simulink model "OPENXWD"  (R2022b)
settings: Solver=ode45  StartTime=0.0  StopTime=inf  RelTol=1e-3  EnableMultiTasking=on
PreLoadFcn:
  | run('Parameters\FSE_Parameters.m')
values from neighbouring files (symbols this model uses):
  g = 9.81    [script.m]    (also in srcipt.m)
  h = 0.25    [script.m]    (also in srcipt.m)
  Ki_pl = 0.01    [srcipt.m]
  Kp_pl = 0.1    [srcipt.m]
  L = 2.6    [script.m]    (also in srcipt.m)
  lf = 2.1    [script.m]    (also in srcipt.m)
  lr = 0.5    [script.m]    (also in srcipt.m)
  ls = 1.242    [script.m]    (also in srcipt.m)
  m = 180    [script.m]    (also in srcipt.m)
  rw = 0.217    [script.m]    (also in srcipt.m)
  Ts = 0.01    [srcipt.m]
undefined symbols (not defined in the file or in its folder): c, gain, Ku, l_ESO, min_yaw_rate
libraries: CarMaker4SL x45, simulink x9
(part 3 of 3)

== system OPENXWD/CarMaker/IPG Vehicle/PowerTrain/TorqueVectoring/Torque distribution/T_FR1 ==
  FzRR : Inport
  Tt : Inport  Port=2
  ^Mz : Inport  Port=3
  Gain : Gain  Gain=rw/ls
  Gain1 : Gain  Gain=1/(m*g)
  Product : Product
  Sum : Sum
  T_RR : Outport
  wires:
  Gain/1 -> Sum/2
  Tt/1 -> Sum/1
  ^Mz/1 -> Gain/1
  FzRR/1 -> Gain1/1
  Gain1/1 -> Product/1
  Product/1 -> T_RR/1
  Sum/1 -> Product/2

== system OPENXWD/CarMaker/IPG Vehicle/PowerTrain/TorqueVectoring/Torque distribution/T_RL ==
  FzRL : Inport
  Tt : Inport  Port=2
  ^Mz : Inport  Port=3
  Gain : Gain  Gain=rw/ls
  Gain1 : Gain  Gain=1/(m*g)
  Product : Product
  Sum : Sum  Inputs=+-
  T_RL : Outport
  wires:
  Gain/1 -> Sum/2
  Tt/1 -> Sum/1
  ^Mz/1 -> Gain/1
  FzRL/1 -> Gain1/1
  Gain1/1 -> Product/1
  Product/1 -> T_RL/1
  Sum/1 -> Product/2

== system OPENXWD/CarMaker/IPG Vehicle/TV/TorqueVectoring/Torque distribution/Fzfl ==
  ax : Inport
  ay : Inport  Port=2
  Constant : Constant  Value=g*lr
  Gain : Gain  Gain=m/(2*L)
  Gain1 : Gain  Gain=h
  Gain2 : Gain  Gain=(h*lr)/(ls)
  Sum : Sum  Inputs=+--
  Fzfl : Outport
  wires:
  Sum/1 -> Gain/1
  Constant/1 -> Sum/1
  Gain1/1 -> Sum/2
  ax/1 -> Gain1/1
  ay/1 -> Gain2/1
  Gain2/1 -> Sum/3
  Gain/1 -> Fzfl/1

== system OPENXWD/CarMaker/IPG Vehicle/TV/TorqueVectoring/Torque distribution/Fzfr ==
  ay : Inport
  ax : Inport  Port=2
  Constant : Constant  Value=g*lr
  Gain : Gain  Gain=m/(2*L)
  Gain1 : Gain  Gain=h
  Gain2 : Gain  Gain=(h*lr)/(ls)
  Sum : Sum  Inputs=+-+
  Fzfr : Outport
  wires:
  Sum/1 -> Gain/1
  Constant/1 -> Sum/1
  Gain1/1 -> Sum/2
  ax/1 -> Gain1/1
  ay/1 -> Gain2/1
  Gain2/1 -> Sum/3
  Gain/1 -> Fzfr/1

== system OPENXWD/CarMaker/IPG Vehicle/TV/TorqueVectoring/Torque distribution/Fzrl ==
  ax : Inport
  ay : Inport  Port=2
  Constant : Constant  Value=g*lf
  Gain : Gain  Gain=m/(2*L)
  Gain1 : Gain  Gain=h
  Gain2 : Gain  Gain=(h*lf)/(ls)
  Sum : Sum  Inputs=++-
  Fzrl : Outport
  wires:
  Gain/1 -> Fzrl/1
  Gain2/1 -> Sum/3
  ay/1 -> Gain2/1
  Sum/1 -> Gain/1
  Constant/1 -> Sum/1
  ax/1 -> Gain1/1
  Gain1/1 -> Sum/2

== system OPENXWD/CarMaker/IPG Vehicle/TV/TorqueVectoring/Torque distribution/Fzrr ==
  ay : Inport
  ax : Inport  Port=2
  Constant : Constant  Value=g*lf
  Gain : Gain  Gain=m/(2*L)
  Gain1 : Gain  Gain=h
  Gain2 : Gain  Gain=(h*lf)/(ls)
  Sum : Sum  Inputs=+++
  Fzrr : Outport
  wires:
  Gain/1 -> Fzrr/1
  Gain2/1 -> Sum/3
  ay/1 -> Gain2/1
  Sum/1 -> Gain/1
  Constant/1 -> Sum/1
  ax/1 -> Gain1/1
  Gain1/1 -> Sum/2

== system OPENXWD/CarMaker/IPG Vehicle/TV/TorqueVectoring/Torque distribution/Regulator ==
  User input : Inport
  Rear wheels speed : Inport  Port=2
  Vehicle speed : Inport  Port=3
  Constant : Constant  Value=0.1175
  Constant1 : Constant  Value=0
  Feedback controler : Subsystem
  Govenor : Subsystem
  Power Limiting : Subsystem
  Saturation Dynamic : simulink/Discontinuities/Saturation Dynamic  OutMin=[]  OutMax=[]  OutDataTypeStr=Inherit: Same as second input  OutDataType=fixdt(1, 16)  OutScaling=2^-10  DoSatur=off
  Sum : Sum  Inputs=|+-
  Zero-Order Hold : ZeroOrderHold  SampleTime=c.Ts
  demanded torque : Outport
  wires:
  Zero-Order Hold/1 -> Feedback controler/1(e)
  Rear wheels speed/1 -> Power Limiting/1(rear wheel speed), Sum/2  "rear_wheel_speed[m/s]"
  Sum/1 -> Zero-Order Hold/1  "e_wheels_speed[m/s]"
  Constant/1 -> Govenor/1(Ref slip ratio)
  Govenor/1(velocity) -> Sum/1  "ref_v_R [m/s]"
  User input/1 -> Feedback controler/2(User input)
  Vehicle speed/1 -> Govenor/2(vehicle speed)
  Saturation Dynamic/1 -> demanded torque/1, Feedback controler/3(u_now)
  Feedback controler/1(demanded torque) -> Saturation Dynamic/2
  Constant1/1 -> Saturation Dynamic/3
  Power Limiting/1(Out1) -> Saturation Dynamic/1  "torque_power_limiting[Nm]"

== system OPENXWD/CarMaker/IPG Vehicle/TV/TorqueVectoring/Torque distribution/Regulator1 ==
  User input : Inport
  Rear wheels speed : Inport  Port=2
  Vehicle speed : Inport  Port=3
  Constant : Constant  Value=0.1175
  Constant1 : Constant  Value=0
  Feedback controler : Subsystem
  Govenor : Subsystem
  Power Limiting : Subsystem
  Saturation Dynamic : simulink/Discontinuities/Saturation Dynamic  OutMin=[]  OutMax=[]  OutDataTypeStr=Inherit: Same as second input  OutDataType=fixdt(1, 16)  OutScaling=2^-10  DoSatur=off
  Sum : Sum  Inputs=|+-
  Zero-Order Hold : ZeroOrderHold  SampleTime=c.Ts
  demanded torque : Outport
  wires:
  Zero-Order Hold/1 -> Feedback controler/1(e)
  Rear wheels speed/1 -> Power Limiting/1(rear wheel speed), Sum/2  "rear_wheel_speed[m/s]"
  Sum/1 -> Zero-Order Hold/1  "e_wheels_speed[m/s]"
  Constant/1 -> Govenor/1(Ref slip ratio)
  Govenor/1(velocity) -> Sum/1  "ref_v_R [m/s]"
  User input/1 -> Feedback controler/2(User input)
  Vehicle speed/1 -> Govenor/2(vehicle speed)
  Saturation Dynamic/1 -> demanded torque/1, Feedback controler/3(u_now)
  Feedback controler/1(demanded torque) -> Saturation Dynamic/2
  Constant1/1 -> Saturation Dynamic/3
  Power Limiting/1(Out1) -> Saturation Dynamic/1  "torque_power_limiting[Nm]"

== system OPENXWD/CarMaker/IPG Vehicle/TV/TorqueVectoring/Torque distribution/Regulator2 ==
  User input : Inport
  Rear wheels speed : Inport  Port=2
  Vehicle speed : Inport  Port=3
  Constant : Constant  Value=0.1175
  Constant1 : Constant  Value=0
  Feedback controler : Subsystem
  Govenor : Subsystem
  Power Limiting : Subsystem
  Saturation Dynamic : simulink/Discontinuities/Saturation Dynamic  OutMin=[]  OutMax=[]  OutDataTypeStr=Inherit: Same as second input  OutDataType=fixdt(1, 16)  OutScaling=2^-10  DoSatur=off
  Sum : Sum  Inputs=|+-
  Zero-Order Hold : ZeroOrderHold  SampleTime=c.Ts
  demanded torque : Outport
  wires:
  Zero-Order Hold/1 -> Feedback controler/1(e)
  Rear wheels speed/1 -> Power Limiting/1(rear wheel speed), Sum/2  "rear_wheel_speed[m/s]"
  Sum/1 -> Zero-Order Hold/1  "e_wheels_speed[m/s]"
  Constant/1 -> Govenor/1(Ref slip ratio)
  Govenor/1(velocity) -> Sum/1  "ref_v_R [m/s]"
  User input/1 -> Feedback controler/2(User input)
  Vehicle speed/1 -> Govenor/2(vehicle speed)
  Saturation Dynamic/1 -> demanded torque/1, Feedback controler/3(u_now)
  Feedback controler/1(demanded torque) -> Saturation Dynamic/2
  Constant1/1 -> Saturation Dynamic/3
  Power Limiting/1(Out1) -> Saturation Dynamic/1  "torque_power_limiting[Nm]"

== system OPENXWD/CarMaker/IPG Vehicle/TV/TorqueVectoring/Torque distribution/Regulator3 ==
  User input : Inport
  Rear wheels speed : Inport  Port=2
  Vehicle speed : Inport  Port=3
  Constant : Constant  Value=0.1175
  Constant1 : Constant  Value=0
  Feedback controler : Subsystem
  Govenor : Subsystem
  Power Limiting : Subsystem
  Saturation Dynamic : simulink/Discontinuities/Saturation Dynamic  OutMin=[]  OutMax=[]  OutDataTypeStr=Inherit: Same as second input  OutDataType=fixdt(1, 16)  OutScaling=2^-10  DoSatur=off
  Sum : Sum  Inputs=|+-
  Zero-Order Hold : ZeroOrderHold  SampleTime=c.Ts
  demanded torque : Outport
  wires:
  Zero-Order Hold/1 -> Feedback controler/1(e)
  Rear wheels speed/1 -> Power Limiting/1(rear wheel speed), Sum/2  "rear_wheel_speed[m/s]"
  Sum/1 -> Zero-Order Hold/1  "e_wheels_speed[m/s]"
  Constant/1 -> Govenor/1(Ref slip ratio)
  Govenor/1(velocity) -> Sum/1  "ref_v_R [m/s]"
  User input/1 -> Feedback controler/2(User input)
  Vehicle speed/1 -> Govenor/2(vehicle speed)
  Saturation Dynamic/1 -> demanded torque/1, Feedback controler/3(u_now)
  Feedback controler/1(demanded torque) -> Saturation Dynamic/2
  Constant1/1 -> Saturation Dynamic/3
  Power Limiting/1(Out1) -> Saturation Dynamic/1  "torque_power_limiting[Nm]"

== system OPENXWD/CarMaker/IPG Vehicle/TV/TorqueVectoring/Torque distribution/T_FL ==
  Fzfl : Inport
  Tt : Inport  Port=2
  ^Mz : Inport  Port=3
  Gain : Gain  Gain=rw/ls
  Gain1 : Gain  Gain=1/(m*g)
  Product : Product
  Sum : Sum  Inputs=+-
  T_FL : Outport
  wires:
  Gain/1 -> Sum/2
  Tt/1 -> Sum/1
  ^Mz/1 -> Gain/1
  Fzfl/1 -> Gain1/1
  Gain1/1 -> Product/1
  Product/1 -> T_FL/1
  Sum/1 -> Product/2

== system OPENXWD/CarMaker/IPG Vehicle/TV/TorqueVectoring/Torque distribution/T_FR ==
  Fzfr : Inport
  Tt : Inport  Port=2
  ^Mz : Inport  Port=3
  Gain : Gain  Gain=rw/ls
  Gain1 : Gain  Gain=1/(m*g)
  Product : Product
  Sum : Sum
  T_FR : Outport
  wires:
  Gain/1 -> Sum/2
  Tt/1 -> Sum/1
  ^Mz/1 -> Gain/1
  Fzfr/1 -> Gain1/1
  Gain1/1 -> Product/1
  Product/1 -> T_FR/1
  Sum/1 -> Product/2

== system OPENXWD/CarMaker/IPG Vehicle/TV/TorqueVectoring/Torque distribution/T_RL ==
  FzRL : Inport
  Tt : Inport  Port=2
  ^Mz : Inport  Port=3
  Gain : Gain  Gain=rw/ls
  Gain1 : Gain  Gain=1/(m*g)
  Product : Product
  Sum : Sum  Inputs=+-
  T_RL : Outport
  wires:
  Gain/1 -> Sum/2
  Tt/1 -> Sum/1
  ^Mz/1 -> Gain/1
  FzRL/1 -> Gain1/1
  Gain1/1 -> Product/1
  Product/1 -> T_RL/1
  Sum/1 -> Product/2

== system OPENXWD/CarMaker/IPG Vehicle/TV/TorqueVectoring/Torque distribution/T_RR ==
  FzRR : Inport
  Tt : Inport  Port=2
  ^Mz : Inport  Port=3
  Gain : Gain  Gain=rw/ls
  Gain1 : Gain  Gain=1/(m*g)
  Product : Product
  Sum : Sum
  T_RR : Outport
  wires:
  Gain/1 -> Sum/2
  Tt/1 -> Sum/1
  ^Mz/1 -> Gain/1
  FzRR/1 -> Gain1/1
  Gain1/1 -> Product/1
  Product/1 -> T_RR/1
  Sum/1 -> Product/2

== system OPENXWD/CarMaker/IPG Vehicle/The Best TorqueVectoring/TorqueVectoring/Torque distribution Tv/Fzfl ==
  ax : Inport
  ay : Inport  Port=2
  Constant : Constant  Value=g*lr
  Gain : Gain  Gain=m/(2*L)
  Gain1 : Gain  Gain=h
  Gain2 : Gain  Gain=(h*lr)/(ls)
  Sum : Sum  Inputs=+--
  Fzfl : Outport
  wires:
  Sum/1 -> Gain/1
  Constant/1 -> Sum/1
  Gain1/1 -> Sum/2
  ax/1 -> Gain1/1
  ay/1 -> Gain2/1
  Gain2/1 -> Sum/3
  Gain/1 -> Fzfl/1

== system OPENXWD/CarMaker/IPG Vehicle/The Best TorqueVectoring/TorqueVectoring/Torque distribution Tv/Fzfr ==
  ay : Inport
  ax : Inport  Port=2
  Constant : Constant  Value=g*lr
  Gain : Gain  Gain=m/(2*L)
  Gain1 : Gain  Gain=h
  Gain2 : Gain  Gain=(h*lr)/(ls)
  Sum : Sum  Inputs=+-+
  Fzfr : Outport
  wires:
  Sum/1 -> Gain/1
  Constant/1 -> Sum/1
  Gain1/1 -> Sum/2
  ax/1 -> Gain1/1
  ay/1 -> Gain2/1
  Gain2/1 -> Sum/3
  Gain/1 -> Fzfr/1

== system OPENXWD/CarMaker/IPG Vehicle/The Best TorqueVectoring/TorqueVectoring/Torque distribution Tv/Fzrl ==
  ax : Inport
  ay : Inport  Port=2
  Constant : Constant  Value=g*lf
  Gain : Gain  Gain=m/(2*L)
  Gain1 : Gain  Gain=h
  Gain2 : Gain  Gain=(h*lf)/(ls)
  Sum : Sum  Inputs=++-
  Fzrl : Outport
  wires:
  Gain/1 -> Fzrl/1
  Gain2/1 -> Sum/3
  ay/1 -> Gain2/1
  Sum/1 -> Gain/1
  Constant/1 -> Sum/1
  ax/1 -> Gain1/1
  Gain1/1 -> Sum/2

== system OPENXWD/CarMaker/IPG Vehicle/The Best TorqueVectoring/TorqueVectoring/Torque distribution Tv/Fzrr ==
  ay : Inport
  ax : Inport  Port=2
  Constant : Constant  Value=g*lf
  Gain : Gain  Gain=m/(2*L)
  Gain1 : Gain  Gain=h
  Gain2 : Gain  Gain=(h*lf)/(ls)
  Sum : Sum  Inputs=+++
  Fzrr : Outport
  wires:
  Gain/1 -> Fzrr/1
  Gain2/1 -> Sum/3
  ay/1 -> Gain2/1
  Sum/1 -> Gain/1
  Constant/1 -> Sum/1
  ax/1 -> Gain1/1
  Gain1/1 -> Sum/2

== system OPENXWD/CarMaker/IPG Vehicle/The Best TorqueVectoring/TorqueVectoring/Torque distribution Tv/T_FL ==
  Fzfl : Inport
  Tt : Inport  Port=2
  ^Mz : Inport  Port=3
  Gain : Gain  Gain=rw/ls
  Gain1 : Gain  Gain=1/(m*g)
  Product : Product
  Sum : Sum  Inputs=+-
  T_FL : Outport
  wires:
  Gain/1 -> Sum/2
  Tt/1 -> Sum/1
  ^Mz/1 -> Gain/1
  Fzfl/1 -> Gain1/1
  Gain1/1 -> Product/1
  Product/1 -> T_FL/1
  Sum/1 -> Product/2

== system OPENXWD/CarMaker/IPG Vehicle/The Best TorqueVectoring/TorqueVectoring/Torque distribution Tv/T_FR ==
  Fzfr : Inport
  Tt : Inport  Port=2
  ^Mz : Inport  Port=3
  Gain : Gain  Gain=rw/ls
  Gain1 : Gain  Gain=1/(m*g)
  Product : Product
  Sum : Sum
  T_FR : Outport
  wires:
  Gain/1 -> Sum/2
  Tt/1 -> Sum/1
  ^Mz/1 -> Gain/1
  Fzfr/1 -> Gain1/1
  Gain1/1 -> Product/1
  Product/1 -> T_FR/1
  Sum/1 -> Product/2

== system OPENXWD/CarMaker/IPG Vehicle/The Best TorqueVectoring/TorqueVectoring/Torque distribution Tv/T_FR1 ==
  FzRR : Inport
  Tt : Inport  Port=2
  ^Mz : Inport  Port=3
  Gain : Gain  Gain=rw/ls
  Gain1 : Gain  Gain=1/(m*g)
  Product : Product
  Sum : Sum
  T_RR : Outport
  wires:
  Gain/1 -> Sum/2
  Tt/1 -> Sum/1
  ^Mz/1 -> Gain/1
  FzRR/1 -> Gain1/1
  Gain1/1 -> Product/1
  Product/1 -> T_RR/1
  Sum/1 -> Product/2

== system OPENXWD/CarMaker/IPG Vehicle/The Best TorqueVectoring/TorqueVectoring/Torque distribution Tv/T_RL ==
  FzRL : Inport
  Tt : Inport  Port=2
  ^Mz : Inport  Port=3
  Gain : Gain  Gain=rw/ls
  Gain1 : Gain  Gain=1/(m*g)
  Product : Product
  Sum : Sum  Inputs=+-
  T_RL : Outport
  wires:
  Gain/1 -> Sum/2
  Tt/1 -> Sum/1
  ^Mz/1 -> Gain/1
  FzRL/1 -> Gain1/1
  Gain1/1 -> Product/1
  Product/1 -> T_RL/1
  Sum/1 -> Product/2

== system OPENXWD/CarMaker/IPG Vehicle/TorqueVectoring/TorqueVectoring/Torque distribution/Fzfl ==
  ax : Inport
  ay : Inport  Port=2
  Constant : Constant  Value=g*lr
  Gain : Gain  Gain=m/(2*L)
  Gain1 : Gain  Gain=h
  Gain2 : Gain  Gain=(h*lr)/(ls)
  Sum : Sum  Inputs=+--
  Fzfl : Outport
  wires:
  Sum/1 -> Gain/1
  Constant/1 -> Sum/1
  Gain1/1 -> Sum/2
  ax/1 -> Gain1/1
  ay/1 -> Gain2/1
  Gain2/1 -> Sum/3
  Gain/1 -> Fzfl/1

== system OPENXWD/CarMaker/IPG Vehicle/TorqueVectoring/TorqueVectoring/Torque distribution/Fzfr ==
  ay : Inport
  ax : Inport  Port=2
  Constant : Constant  Value=g*lr
  Gain : Gain  Gain=m/(2*L)
  Gain1 : Gain  Gain=h
  Gain2 : Gain  Gain=(h*lr)/(ls)
  Sum : Sum  Inputs=+-+
  Fzfr : Outport
  wires:
  Sum/1 -> Gain/1
  Constant/1 -> Sum/1
  Gain1/1 -> Sum/2
  ax/1 -> Gain1/1
  ay/1 -> Gain2/1
  Gain2/1 -> Sum/3
  Gain/1 -> Fzfr/1

== system OPENXWD/CarMaker/IPG Vehicle/TorqueVectoring/TorqueVectoring/Torque distribution/Fzrl ==
  ax : Inport
  ay : Inport  Port=2
  Constant : Constant  Value=g*lf
  Gain : Gain  Gain=m/(2*L)
  Gain1 : Gain  Gain=h
  Gain2 : Gain  Gain=(h*lf)/(ls)
  Sum : Sum  Inputs=++-
  Fzrl : Outport
  wires:
  Gain/1 -> Fzrl/1
  Gain2/1 -> Sum/3
  ay/1 -> Gain2/1
  Sum/1 -> Gain/1
  Constant/1 -> Sum/1
  ax/1 -> Gain1/1
  Gain1/1 -> Sum/2

== system OPENXWD/CarMaker/IPG Vehicle/TorqueVectoring/TorqueVectoring/Torque distribution/Fzrr ==
  ay : Inport
  ax : Inport  Port=2
  Constant : Constant  Value=g*lf
  Gain : Gain  Gain=m/(2*L)
  Gain1 : Gain  Gain=h
  Gain2 : Gain  Gain=(h*lf)/(ls)
  Sum : Sum  Inputs=+++
  Fzrr : Outport
  wires:
  Gain/1 -> Fzrr/1
  Gain2/1 -> Sum/3
  ay/1 -> Gain2/1
  Sum/1 -> Gain/1
  Constant/1 -> Sum/1
  ax/1 -> Gain1/1
  Gain1/1 -> Sum/2

== system OPENXWD/CarMaker/IPG Vehicle/TorqueVectoring/TorqueVectoring/Torque distribution/T_FL ==
  Fzfl : Inport
  Tt : Inport  Port=2
  ^Mz : Inport  Port=3
  Gain : Gain  Gain=rw/ls
  Gain1 : Gain  Gain=1/(m*g)
  Product : Product
  Sum : Sum  Inputs=+-
  T_FL : Outport
  wires:
  Gain/1 -> Sum/2
  Tt/1 -> Sum/1
  ^Mz/1 -> Gain/1
  Fzfl/1 -> Gain1/1
  Gain1/1 -> Product/1
  Product/1 -> T_FL/1
  Sum/1 -> Product/2

== system OPENXWD/CarMaker/IPG Vehicle/TorqueVectoring/TorqueVectoring/Torque distribution/T_FR ==
  Fzfr : Inport
  Tt : Inport  Port=2
  ^Mz : Inport  Port=3
  Gain : Gain  Gain=rw/ls
  Gain1 : Gain  Gain=1/(m*g)
  Product : Product
  Sum : Sum
  T_FR : Outport
  wires:
  Gain/1 -> Sum/2
  Tt/1 -> Sum/1
  ^Mz/1 -> Gain/1
  Fzfr/1 -> Gain1/1
  Gain1/1 -> Product/1
  Product/1 -> T_FR/1
  Sum/1 -> Product/2

== system OPENXWD/CarMaker/IPG Vehicle/TorqueVectoring/TorqueVectoring/Torque distribution/T_FR1 ==
  FzRR : Inport
  Tt : Inport  Port=2
  ^Mz : Inport  Port=3
  Gain : Gain  Gain=rw/ls
  Gain1 : Gain  Gain=1/(m*g)
  Product : Product
  Sum : Sum
  T_RR : Outport
  wires:
  Gain/1 -> Sum/2
  Tt/1 -> Sum/1
  ^Mz/1 -> Gain/1
  FzRR/1 -> Gain1/1
  Gain1/1 -> Product/1
  Product/1 -> T_RR/1
  Sum/1 -> Product/2

== system OPENXWD/CarMaker/IPG Vehicle/TorqueVectoring/TorqueVectoring/Torque distribution/T_RL ==
  FzRL : Inport
  Tt : Inport  Port=2
  ^Mz : Inport  Port=3
  Gain : Gain  Gain=rw/ls
  Gain1 : Gain  Gain=1/(m*g)
  Product : Product
  Sum : Sum  Inputs=+-
  T_RL : Outport
  wires:
  Gain/1 -> Sum/2
  Tt/1 -> Sum/1
  ^Mz/1 -> Gain/1
  FzRL/1 -> Gain1/1
  Gain1/1 -> Product/1
  Product/1 -> T_RL/1
  Sum/1 -> Product/2

== system OPENXWD/CarMaker/IPG Vehicle/TV/TorqueVectoring/Torque distribution/Regulator/Feedback controler ==
  note: u_sat
  e : Inport
  User input : Inport  Port=2
  u_now : Inport  Port=3
  Constant : Constant  Value=0
  Constant1 : Constant  Value=l_ESO
  Constant3 : Constant  Value=gain
  MATLAB Function : MATLAB Function  TreatAsAtomicUnit=on
  MATLAB Function1 : MATLAB Function  TreatAsAtomicUnit=on
  Saturation Dynamic : simulink/Discontinuities/Saturation Dynamic  OutMin=[]  OutMax=[]  OutDataTypeStr=Inherit: Same as second input  OutDataType=fixdt(1, 16)  OutScaling=2^-10  DoSatur=off
  Unit Delay : UnitDelay  InitialCondition=[0;0]  SampleTime=0.002  HasFrameUpgradeWarning=on
  Unit Delay1 : UnitDelay  SampleTime=0.002  HasFrameUpgradeWarning=on
  Unit Delay2 : UnitDelay  SampleTime=c.inv_delay  HasFrameUpgradeWarning=on
  demanded torque : Outport
  wires:
  e/1 -> MATLAB Function/1(e), MATLAB Function1/1(e)
  Unit Delay/1 -> MATLAB Function1/3(x_hat)
  MATLAB Function/1(y) -> Saturation Dynamic/2
  Saturation Dynamic/1 -> demanded torque/1
  User input/1 -> Saturation Dynamic/1
  Constant/1 -> Saturation Dynamic/3
  u_now/1 -> Unit Delay1/1
  MATLAB Function1/1(F_hat) -> MATLAB Function/2(F)  "F_hat"
  MATLAB Function1/2(x_hat_k_1) -> Unit Delay/1
  Constant1/1 -> MATLAB Function1/4(l_ESO)
  Constant3/1 -> MATLAB Function/3(k)
  Unit Delay1/1 -> Unit Delay2/1
  Unit Delay2/1 -> MATLAB Function1/2(u)

== system OPENXWD/CarMaker/IPG Vehicle/TV/TorqueVectoring/Torque distribution/Regulator/Govenor ==
  Ref slip ratio : Inport
  vehicle speed : Inport  Port=2
  Constant : Constant
  Divide : Product  Inputs=*/
  Gain : Gain  Gain=-1
  Max : MinMax  Function=max  Inputs=2
  Min ref rear wheel speed to prevent stopping at 0 m/s : Constant  Value=c.min_ref_speed
  Sum : Sum  Inputs=|-+
  velocity : Outport
  wires:
  Ref slip ratio/1 -> Sum/2
  Constant/1 -> Sum/1
  Max/1 -> velocity/1
  Min ref rear wheel speed to prevent stopping at 0 m/s/1 -> Max/2
  vehicle speed/1 -> Divide/1
  Sum/1 -> Divide/2
  Gain/1 -> Max/1
  Divide/1 -> Gain/1

== system OPENXWD/CarMaker/IPG Vehicle/TV/TorqueVectoring/Torque distribution/Regulator/Power Limiting ==
  note: P = T * gr * omega
      | Tmax = P / gr / omega * (efficiency + safe factor)
  rear wheel speed : Inport
  Abs : Abs  SaturateOnIntegerOverflow=off
  Constant : Constant  Value=20000
  Constant2 : Constant  Value=1/c.G_R/c.r_dyn * (1 / c.inv_motor_efficiency + c.power_limit_safe_factor)
  Constant3 : Constant  Value=5
  Divide : Product  Inputs=*/
  Divide1 : Product  Inputs=*/
  Switch : Switch  Criteria=u2 > Threshold  Threshold=10  SaturateOnIntegerOverflow=off  InputSameDT=off
  Out1 : Outport
  wires:
  Divide/1 -> Divide1/1
  Switch/1 -> Divide/2
  Constant3/1 -> Switch/3
  Constant2/1 -> Divide1/2
  rear wheel speed/1 -> Switch/1, Switch/2
  Constant/1 -> Out1/1, Divide/1
  Divide1/1 -> Abs/1

== system OPENXWD/CarMaker/IPG Vehicle/TV/TorqueVectoring/Torque distribution/Regulator1/Feedback controler ==
  note: u_sat
  e : Inport
  User input : Inport  Port=2
  u_now : Inport  Port=3
  Constant : Constant  Value=0
  Constant1 : Constant  Value=l_ESO
  Constant3 : Constant  Value=gain
  MATLAB Function : MATLAB Function  TreatAsAtomicUnit=on
  MATLAB Function1 : MATLAB Function  TreatAsAtomicUnit=on
  Saturation Dynamic : simulink/Discontinuities/Saturation Dynamic  OutMin=[]  OutMax=[]  OutDataTypeStr=Inherit: Same as second input  OutDataType=fixdt(1, 16)  OutScaling=2^-10  DoSatur=off
  Unit Delay : UnitDelay  InitialCondition=[0;0]  SampleTime=0.002  HasFrameUpgradeWarning=on
  Unit Delay1 : UnitDelay  SampleTime=0.002  HasFrameUpgradeWarning=on
  Unit Delay2 : UnitDelay  SampleTime=c.inv_delay  HasFrameUpgradeWarning=on
  demanded torque : Outport
  wires:
  e/1 -> MATLAB Function/1(e), MATLAB Function1/1(e)
  Unit Delay/1 -> MATLAB Function1/3(x_hat)
  MATLAB Function/1(y) -> Saturation Dynamic/2
  Saturation Dynamic/1 -> demanded torque/1
  User input/1 -> Saturation Dynamic/1
  Constant/1 -> Saturation Dynamic/3
  u_now/1 -> Unit Delay1/1
  MATLAB Function1/1(F_hat) -> MATLAB Function/2(F)  "F_hat"
  MATLAB Function1/2(x_hat_k_1) -> Unit Delay/1
  Constant1/1 -> MATLAB Function1/4(l_ESO)
  Constant3/1 -> MATLAB Function/3(k)
  Unit Delay1/1 -> Unit Delay2/1
  Unit Delay2/1 -> MATLAB Function1/2(u)

== system OPENXWD/CarMaker/IPG Vehicle/TV/TorqueVectoring/Torque distribution/Regulator1/Govenor ==
  Ref slip ratio : Inport
  vehicle speed : Inport  Port=2
  Constant : Constant
  Divide : Product  Inputs=*/
  Gain : Gain  Gain=-1
  Max : MinMax  Function=max  Inputs=2
  Min ref rear wheel speed to prevent stopping at 0 m/s : Constant  Value=c.min_ref_speed
  Sum : Sum  Inputs=|-+
  velocity : Outport
  wires:
  Ref slip ratio/1 -> Sum/2
  Constant/1 -> Sum/1
  Max/1 -> velocity/1
  Min ref rear wheel speed to prevent stopping at 0 m/s/1 -> Max/2
  vehicle speed/1 -> Divide/1
  Sum/1 -> Divide/2
  Gain/1 -> Max/1
  Divide/1 -> Gain/1

== system OPENXWD/CarMaker/IPG Vehicle/TV/TorqueVectoring/Torque distribution/Regulator1/Power Limiting ==
  note: P = T * gr * omega
      | Tmax = P / gr / omega * (efficiency + safe factor)
  rear wheel speed : Inport
  Abs : Abs  SaturateOnIntegerOverflow=off
  Constant : Constant  Value=20000
  Constant2 : Constant  Value=1/c.G_R/c.r_dyn * (1 / c.inv_motor_efficiency + c.power_limit_safe_factor)
  Constant3 : Constant  Value=5
  Divide : Product  Inputs=*/
  Divide1 : Product  Inputs=*/
  Switch : Switch  Criteria=u2 > Threshold  Threshold=10  SaturateOnIntegerOverflow=off  InputSameDT=off
  Out1 : Outport
  wires:
  Divide/1 -> Divide1/1
  Switch/1 -> Divide/2
  Constant3/1 -> Switch/3
  Constant2/1 -> Divide1/2
  rear wheel speed/1 -> Switch/1, Switch/2
  Constant/1 -> Out1/1, Divide/1
  Divide1/1 -> Abs/1

== system OPENXWD/CarMaker/IPG Vehicle/TV/TorqueVectoring/Torque distribution/Regulator2/Feedback controler ==
  note: u_sat
  e : Inport
  User input : Inport  Port=2
  u_now : Inport  Port=3
  Constant : Constant  Value=0
  Constant1 : Constant  Value=l_ESO
  Constant3 : Constant  Value=gain
  MATLAB Function : MATLAB Function  TreatAsAtomicUnit=on
  MATLAB Function1 : MATLAB Function  TreatAsAtomicUnit=on
  Saturation Dynamic : simulink/Discontinuities/Saturation Dynamic  OutMin=[]  OutMax=[]  OutDataTypeStr=Inherit: Same as second input  OutDataType=fixdt(1, 16)  OutScaling=2^-10  DoSatur=off
  Unit Delay : UnitDelay  InitialCondition=[0;0]  SampleTime=0.002  HasFrameUpgradeWarning=on
  Unit Delay1 : UnitDelay  SampleTime=0.002  HasFrameUpgradeWarning=on
  Unit Delay2 : UnitDelay  SampleTime=c.inv_delay  HasFrameUpgradeWarning=on
  demanded torque : Outport
  wires:
  e/1 -> MATLAB Function/1(e), MATLAB Function1/1(e)
  Unit Delay/1 -> MATLAB Function1/3(x_hat)
  MATLAB Function/1(y) -> Saturation Dynamic/2
  Saturation Dynamic/1 -> demanded torque/1
  User input/1 -> Saturation Dynamic/1
  Constant/1 -> Saturation Dynamic/3
  u_now/1 -> Unit Delay1/1
  MATLAB Function1/1(F_hat) -> MATLAB Function/2(F)  "F_hat"
  MATLAB Function1/2(x_hat_k_1) -> Unit Delay/1
  Constant1/1 -> MATLAB Function1/4(l_ESO)
  Constant3/1 -> MATLAB Function/3(k)
  Unit Delay1/1 -> Unit Delay2/1
  Unit Delay2/1 -> MATLAB Function1/2(u)

== system OPENXWD/CarMaker/IPG Vehicle/TV/TorqueVectoring/Torque distribution/Regulator2/Govenor ==
  Ref slip ratio : Inport
  vehicle speed : Inport  Port=2
  Constant : Constant
  Divide : Product  Inputs=*/
  Gain : Gain  Gain=-1
  Max : MinMax  Function=max  Inputs=2
  Min ref rear wheel speed to prevent stopping at 0 m/s : Constant  Value=c.min_ref_speed
  Sum : Sum  Inputs=|-+
  velocity : Outport
  wires:
  Ref slip ratio/1 -> Sum/2
  Constant/1 -> Sum/1
  Max/1 -> velocity/1
  Min ref rear wheel speed to prevent stopping at 0 m/s/1 -> Max/2
  vehicle speed/1 -> Divide/1
  Sum/1 -> Divide/2
  Gain/1 -> Max/1
  Divide/1 -> Gain/1

== system OPENXWD/CarMaker/IPG Vehicle/TV/TorqueVectoring/Torque distribution/Regulator2/Power Limiting ==
  note: P = T * gr * omega
      | Tmax = P / gr / omega * (efficiency + safe factor)
  rear wheel speed : Inport
  Abs : Abs  SaturateOnIntegerOverflow=off
  Constant : Constant  Value=20000
  Constant2 : Constant  Value=1/c.G_R/c.r_dyn * (1 / c.inv_motor_efficiency + c.power_limit_safe_factor)
  Constant3 : Constant  Value=5
  Divide : Product  Inputs=*/
  Divide1 : Product  Inputs=*/
  Switch : Switch  Criteria=u2 > Threshold  Threshold=10  SaturateOnIntegerOverflow=off  InputSameDT=off
  Out1 : Outport
  wires:
  Divide/1 -> Divide1/1
  Switch/1 -> Divide/2
  Constant3/1 -> Switch/3
  Constant2/1 -> Divide1/2
  rear wheel speed/1 -> Switch/1, Switch/2
  Constant/1 -> Out1/1, Divide/1
  Divide1/1 -> Abs/1

== system OPENXWD/CarMaker/IPG Vehicle/TV/TorqueVectoring/Torque distribution/Regulator3/Feedback controler ==
  note: u_sat
  e : Inport
  User input : Inport  Port=2
  u_now : Inport  Port=3
  Constant : Constant  Value=0
  Constant1 : Constant  Value=l_ESO
  Constant3 : Constant  Value=gain
  MATLAB Function : MATLAB Function  TreatAsAtomicUnit=on
  MATLAB Function1 : MATLAB Function  TreatAsAtomicUnit=on
  Saturation Dynamic : simulink/Discontinuities/Saturation Dynamic  OutMin=[]  OutMax=[]  OutDataTypeStr=Inherit: Same as second input  OutDataType=fixdt(1, 16)  OutScaling=2^-10  DoSatur=off
  Unit Delay : UnitDelay  InitialCondition=[0;0]  SampleTime=0.002  HasFrameUpgradeWarning=on
  Unit Delay1 : UnitDelay  SampleTime=0.002  HasFrameUpgradeWarning=on
  Unit Delay2 : UnitDelay  SampleTime=c.inv_delay  HasFrameUpgradeWarning=on
  demanded torque : Outport
  wires:
  e/1 -> MATLAB Function/1(e), MATLAB Function1/1(e)
  Unit Delay/1 -> MATLAB Function1/3(x_hat)
  MATLAB Function/1(y) -> Saturation Dynamic/2
  Saturation Dynamic/1 -> demanded torque/1
  User input/1 -> Saturation Dynamic/1
  Constant/1 -> Saturation Dynamic/3
  u_now/1 -> Unit Delay1/1
  MATLAB Function1/1(F_hat) -> MATLAB Function/2(F)  "F_hat"
  MATLAB Function1/2(x_hat_k_1) -> Unit Delay/1
  Constant1/1 -> MATLAB Function1/4(l_ESO)
  Constant3/1 -> MATLAB Function/3(k)
  Unit Delay1/1 -> Unit Delay2/1
  Unit Delay2/1 -> MATLAB Function1/2(u)

== system OPENXWD/CarMaker/IPG Vehicle/TV/TorqueVectoring/Torque distribution/Regulator3/Govenor ==
  Ref slip ratio : Inport
  vehicle speed : Inport  Port=2
  Constant : Constant
  Divide : Product  Inputs=*/
  Gain : Gain  Gain=-1
  Max : MinMax  Function=max  Inputs=2
  Min ref rear wheel speed to prevent stopping at 0 m/s : Constant  Value=c.min_ref_speed
  Sum : Sum  Inputs=|-+
  velocity : Outport
  wires:
  Ref slip ratio/1 -> Sum/2
  Constant/1 -> Sum/1
  Max/1 -> velocity/1
  Min ref rear wheel speed to prevent stopping at 0 m/s/1 -> Max/2
  vehicle speed/1 -> Divide/1
  Sum/1 -> Divide/2
  Gain/1 -> Max/1
  Divide/1 -> Gain/1

== system OPENXWD/CarMaker/IPG Vehicle/TV/TorqueVectoring/Torque distribution/Regulator3/Power Limiting ==
  note: P = T * gr * omega
      | Tmax = P / gr / omega * (efficiency + safe factor)
  rear wheel speed : Inport
  Abs : Abs  SaturateOnIntegerOverflow=off
  Constant : Constant  Value=20000
  Constant2 : Constant  Value=1/c.G_R/c.r_dyn * (1 / c.inv_motor_efficiency + c.power_limit_safe_factor)
  Constant3 : Constant  Value=5
  Divide : Product  Inputs=*/
  Divide1 : Product  Inputs=*/
  Switch : Switch  Criteria=u2 > Threshold  Threshold=10  SaturateOnIntegerOverflow=off  InputSameDT=off
  Out1 : Outport
  wires:
  Divide/1 -> Divide1/1
  Switch/1 -> Divide/2
  Constant3/1 -> Switch/3
  Constant2/1 -> Divide1/2
  rear wheel speed/1 -> Switch/1, Switch/2
  Constant/1 -> Out1/1, Divide/1
  Divide1/1 -> Abs/1

== matlab function OPENXWD/CarMaker/IPG Vehicle/TorqueVectoring/power_limiter_system/power_limiter/MATLAB Function1 ==
  settings: updateMethod=DISCRETE  sampleTime=Ts
  data: Trq_FL input; Trq_FL_scaled output; Trq_FR input; Trq_RL input; Trq_RR input; omega_FL input; omega_FR input; omega_RL input; omega_RR input; eta input; P_max input; Trq_FR_scaled output; Trq_RL_scaled output; Trq_RR_scaled output; Kp input; Ki input; Ts input
function [Trq_FL_scaled, Trq_FR_scaled, Trq_RL_scaled, Trq_RR_scaled] = ... 
    scaleTorqueToPowerLimit_PI(Trq_FL, Trq_FR, Trq_RL, Trq_RR, ... 
    omega_FL, omega_FR, omega_RL, omega_RR, eta, P_max, Kp, Ki, Ts)
    % Input parameters:
    % Trq_FL, Trq_FR, Trq_RL, Trq_RR - torque on each wheel
    % omega_FL, omega_FR, omega_RL, omega_RR - angular velocity of each wheel
    % eta - motor efficiency
    % P_max - maximum battery power = 79kW
    % Kp - proportional gain
    % Ki - integral gain
    % Ts - sampling time

    persistent integral_error;
    if isempty(integral_error)
        integral_error = 0;
    end

    P_mech_FL = Trq_FL * omega_FL;
    P_mech_FR = Trq_FR * omega_FR;
    P_mech_RL = Trq_RL * omega_RL;
    P_mech_RR = Trq_RR * omega_RR;
    
    P_mech_total = P_mech_FL + P_mech_FR + P_mech_RL + P_mech_RR;
    
    P_el_total = P_mech_total / eta;

    % PI controller
    error = P_max - P_el_total;
    integral_error = integral_error + error * Ts;
    control_signal = Kp * error + Ki * integral_error;


    if control_signal < 0
        scale_factor = 0;
    else
        scale_factor = min(1, control_signal);
    end
    
    Trq_FL_scaled = Trq_FL * scale_factor;
    Trq_FR_scaled = Trq_FR * scale_factor;
    Trq_RL_scaled = Trq_RL * scale_factor;
    Trq_RR_scaled = Trq_RR * scale_factor;
end

== matlab function OPENXWD/CarMaker/IPG Vehicle/TV/TorqueVectoring/Torque distribution/Regulator1/Feedback controler/MATLAB Function ==
  data: y output; e input; F input; k input
function y = psi(e, F, k)
c = const();
y = (k * e + F) / c.b_0 ;
%alfa_0 = 16.5;
%y = 1 / c.b_0 * (abs(e+1)^alfa_0 * sign(e) + F);
end

== matlab function OPENXWD/CarMaker/IPG Vehicle/TV/TorqueVectoring/Torque distribution/Regulator1/Feedback controler/MATLAB Function1 ==
  data: e input; u input; x_hat input; F_hat output; x_hat_k_1 output; l_ESO input
function [F_hat, x_hat_k_1] = ESO(e, u, x_hat, l_ESO)
c = const();
A = [0, 1; 0, 0];
I = eye(2);
x_hat_k_1 = (I + A*c.Ts) * x_hat + c.Ts * [-c.b_0; 0] * u + l_ESO * c.Ts*(e - [1, 0]*x_hat);
F_hat = x_hat(2);
end

== matlab function OPENXWD/CarMaker/IPG Vehicle/TV/TorqueVectoring/Torque distribution/Regulator/Feedback controler/MATLAB Function ==
  data: y output; e input; F input; k input
function y = psi(e, F, k)
c = const();
y = (k * e + F) / c.b_0 ;
%alfa_0 = 16.5;
%y = 1 / c.b_0 * (abs(e+1)^alfa_0 * sign(e) + F);
end

== matlab function OPENXWD/CarMaker/IPG Vehicle/TV/TorqueVectoring/Torque distribution/Regulator2/Feedback controler/MATLAB Function ==
  data: y output; e input; F input; k input
function y = psi(e, F, k)
c = const();
y = (k * e + F) / c.b_0 ;
%alfa_0 = 16.5;
%y = 1 / c.b_0 * (abs(e+1)^alfa_0 * sign(e) + F);
end

== matlab function OPENXWD/CarMaker/IPG Vehicle/TV/TorqueVectoring/Torque distribution/Regulator2/Feedback controler/MATLAB Function1 ==
  data: e input; u input; x_hat input; F_hat output; x_hat_k_1 output; l_ESO input
function [F_hat, x_hat_k_1] = ESO(e, u, x_hat, l_ESO)
c = const();
A = [0, 1; 0, 0];
I = eye(2);
x_hat_k_1 = (I + A*c.Ts) * x_hat + c.Ts * [-c.b_0; 0] * u + l_ESO * c.Ts*(e - [1, 0]*x_hat);
F_hat = x_hat(2);
end

== matlab function OPENXWD/CarMaker/IPG Vehicle/TV/TorqueVectoring/Torque distribution/Regulator/Feedback controler/MATLAB Function1 ==
  data: e input; u input; x_hat input; F_hat output; x_hat_k_1 output; l_ESO input
function [F_hat, x_hat_k_1] = ESO(e, u, x_hat, l_ESO)
c = const();
A = [0, 1; 0, 0];
I = eye(2);
x_hat_k_1 = (I + A*c.Ts) * x_hat + c.Ts * [-c.b_0; 0] * u + l_ESO * c.Ts*(e - [1, 0]*x_hat);
F_hat = x_hat(2);
end

== matlab function OPENXWD/CarMaker/IPG Vehicle/TV/TorqueVectoring/Torque distribution/Regulator3/Feedback controler/MATLAB Function ==
  data: y output; e input; F input; k input
function y = psi(e, F, k)
c = const();
y = (k * e + F) / c.b_0 ;
%alfa_0 = 16.5;
%y = 1 / c.b_0 * (abs(e+1)^alfa_0 * sign(e) + F);
end

== matlab function OPENXWD/CarMaker/IPG Vehicle/TV/TorqueVectoring/Torque distribution/Regulator3/Feedback controler/MATLAB Function1 ==
  data: e input; u input; x_hat input; F_hat output; x_hat_k_1 output; l_ESO input
function [F_hat, x_hat_k_1] = ESO(e, u, x_hat, l_ESO)
c = const();
A = [0, 1; 0, 0];
I = eye(2);
x_hat_k_1 = (I + A*c.Ts) * x_hat + c.Ts * [-c.b_0; 0] * u + l_ESO * c.Ts*(e - [1, 0]*x_hat);
F_hat = x_hat(2);
end
